simulink model "MIL4L3_SW6_V1_20220211"  (R2018b)
settings: Solver=FixedStepAuto  StartTime=0.0  StopTime=inf  FixedStep=0.001  RelTol=1e-3
PreLoadFcn:
  | A0_MILtest;
undefined symbols (not defined in the file or in its folder): Clb_ICADirect_LaneDisp_StateFive, Clb_ICADirect_LaneDisp_StateFour, Clb_ICADirect_LaneDisp_StateOne, Clb_ICADirect_LaneDisp_StateThree, Clb_ICADirect_LaneDisp_StateTwo, Clb_ICADirect_LaneDisp_StateZero, Clb_ICADirect_LaneDispSW, Clb_ICADirect_TrnLghtsCom_Switch, Clb_ICADirect_TrnLghtsCom_Value, Clb_ICADirect_TrnLghtsCrtl_Inhb, IMAP_Clb_ACU_Driver_Belt, IMAP_Clb_ACU_Driver_Belt_Over, IMAP_Clb_ACU_Passenger_Belt, IMAP_Clb_ACU_Passenger_Belt_Over, IMAP_Clb_ACU_RearLeft_Belt, IMAP_Clb_ACU_RearLeft_Belt_Over, IMAP_Clb_ACU_RearMiddle_Belt, IMAP_Clb_ACU_RearMiddle_Belt_Over, IMAP_Clb_ACU_RearRight_Belt, IMAP_Clb_ACU_RearRight_Belt_Over, IMAP_Clb_AEB_Switch, IMAP_Clb_AEB_Switch_Over, IMAP_Clb_ALC_TLC_Mode, IMAP_Clb_ALC_TLC_Mode_Over, IMAP_Clb_BCM_Battery_Voltage, IMAP_Clb_BCM_Battery_Voltage_Over, IMAP_Clb_BCM_BrakeLamp_State, IMAP_Clb_BCM_BrakeLamp_State_Over, IMAP_Clb_BCM_CHMSL_Status, IMAP_Clb_BCM_CHMSL_Status_Over, IMAP_Clb_BCM_Door_Lock_State, IMAP_Clb_BCM_Door_Lock_State_Over, IMAP_Clb_BCM_FrontWiper_State, IMAP_Clb_BCM_FrontWiper_State_Over, IMAP_Clb_BCM_FrontWiper_Switch, IMAP_Clb_BCM_FrontWiper_Switch_Over, IMAP_Clb_BCM_HazardLamp, IMAP_Clb_BCM_HazardLamp_Over, IMAP_Clb_BCM_HazardLamp_Switch, IMAP_Clb_BCM_HazardLamp_Switch_Over, IMAP_Clb_BCM_HighBeam_State, IMAP_Clb_BCM_HighBeam_State_Over, IMAP_Clb_BCM_Ignition_State, IMAP_Clb_BCM_Ignition_State_Over, IMAP_Clb_BCM_IHBC_Enabled, IMAP_Clb_BCM_IHBC_Enabled_Over, IMAP_Clb_BCM_Left_Light, IMAP_Clb_BCM_Left_Light_Over, IMAP_Clb_BCM_LeftTurn_Switch, IMAP_Clb_BCM_LeftTurn_Switch_Over, IMAP_Clb_BCM_LF_Door_State, IMAP_Clb_BCM_LF_Door_State_Over, IMAP_Clb_BCM_LowBeam_State, IMAP_Clb_BCM_LowBeam_State_Over, IMAP_Clb_BCM_LR_Door_State, IMAP_Clb_BCM_LR_Door_State_Over, IMAP_Clb_BCM_RF_Door_State, IMAP_Clb_BCM_RF_Door_State_Over, IMAP_Clb_BCM_Right_Light, IMAP_Clb_BCM_Right_Light_Over ... (+547)
libraries: CarMaker4SL x2153, simulink x292, dspstat3 x3, canmsglib x2, simulink_extras x1
(part 42 of 52)

== system MIL4L3_SW6_V1_20220211/CarMaker/VehicleControl/OMAP/OMAP1/Runnable_OMAP_10ms_sys/OMAP_Module/ACCS_Direct/ACCS_Define/ACC_State_Synthesis(ACC_SS)/If Action Subsystem3 ==
  ACT_Control_Signal : Inport
  Action Port : ActionPort  InitializeStates=reset  ActionType=else
  Bus Creator : BusCreator  Inputs=15
  Bus Selector1 : BusSelector  OutputSignals=ACCSve_g_ACC_TqReq_convert,ACCSve_d_ACC_TqFlag_convert,ACCSve_g_ACC_DecReq_convert,ACCSve_d_ACC_DecFlag_convert,ACCSve_d_ACC_State_convert,ACCSve_d_ACC_ESCDriveOff_convert,ACCSve_d_ACC_ESCHoldReq_convert,ACCSve_d_ACC_EPBReq_convert
  Constant5 : Constant  Value=0  OutDataTypeStr=uint8
  Data Type Conversion{,1..6} (7 alike) : DataTypeConversion  OutDataTypeStr=uint8
  Gain : Gain  OutDataTypeStr=single
  Signal Conversion : SignalConversion  OverrideOpt=off
  Subsystem : Subsystem
  Subsystem1 : Subsystem
  Subsystem2 : Subsystem
  Subsystem3 : Subsystem
  Subsystem5 : Subsystem
  Subsystem6 : Subsystem
  Control_Ouput : Outport
  wires:
  Bus Selector1/4 -> [ESC_Enable]  "<ACCSve_d_ACC_DecFlag_convert>"
  Bus Selector1/3 -> [ESC_DecTar]  "<ACCSve_g_ACC_DecReq_convert>"
  Bus Selector1/2 -> [EMS_Enable]  "<ACCSve_d_ACC_TqFlag_convert>"
  Bus Selector1/1 -> [EMS_DecTar]  "<ACCSve_g_ACC_TqReq_convert>"
  Data Type Conversion2/1 -> Bus Creator/11  "MDD_deceleration_type"
  Data Type Conversion1/1 -> Bus Creator/10  "MDD_Decelerationcontrol_request"
  Data Type Conversion/1 -> Bus Creator/8  "Powertrain_torquewheel_request"
  Subsystem6/1(TYPE_RAPPORT) -> Bus Creator/9  "TYPE_RAPPORT"
  [EMS_Enable] -> Data Type Conversion/1
  Signal Conversion/1 -> Control_Ouput/1
  Constant5/1 -> Bus Creator/12  "Power_steering_power_cut3F2"
  Gain/1 -> Bus Creator/5  "PotACCTqReq"
  [EMS_Enable] -> Subsystem5/2(In2)
  [EMS_DecTar] -> Subsystem5/1(In1)
  Subsystem3/1(Function_Acc_status) -> Bus Creator/6  "Function_Acc_status"
  Bus Selector1/5 -> Data Type Conversion3/1  "<ACCSve_d_ACC_State_convert>"
  Subsystem2/1(StAcvTqWhlPTPotReq) -> Bus Creator/4  "StAcvTqWhlPTPotReq"
  [ESC_Enable] -> Subsystem2/2(In2)
  Subsystem1/1(TminUpGear) -> Bus Creator/3  "TminUpGear"
  Subsystem/1(TminDownGear) -> Bus Creator/2  "TminDownGear"
  [EMS_Enable] -> Subsystem1/1(In1), Subsystem/1(In1), Subsystem2/1(In1)
  ACT_Control_Signal/1 -> Bus Selector1/1
  Bus Creator/1 -> Signal Conversion/1
  [ESC_DecTar] -> Bus Creator/1  "Deceleration_setpoint_device"
  [EMS_DecTar] -> Gain/1, Bus Creator/7  "ACCTqReq"
  [ESC_Enable] -> Data Type Conversion1/1
  [ESC_Enable] -> Data Type Conversion2/1
  Data Type Conversion3/1 -> Subsystem3/1(In1)
  [ESC_Hold] -> Data Type Conversion5/1
  [ESC_EPB] -> Data Type Conversion6/1
  [ESC_DriveOff] -> Data Type Conversion4/1
  Bus Selector1/6 -> [ESC_DriveOff]  "<ACCSve_d_ACC_ESCDriveOff_convert>"
  Bus Selector1/7 -> [ESC_Hold]  "<ACCSve_d_ACC_ESCHoldReq_convert>"
  Bus Selector1/8 -> [ESC_EPB]  "<ACCSve_d_ACC_EPBReq_convert>"
  Data Type Conversion4/1 -> Bus Creator/13  "OMAPve_y_ADAS_ESCDriveOff"
  Data Type Conversion5/1 -> Bus Creator/14  "OMAPve_y_ADAS_ESCHoldReq"
  Data Type Conversion6/1 -> Bus Creator/15  "OMAPve_y_ADAS_ACCRequestEPB"

== system MIL4L3_SW6_V1_20220211/CarMaker/VehicleControl/OMAP/OMAP1/Runnable_OMAP_10ms_sys/OMAP_Module/ACCS_Direct/ACCS_Define/Human_Machine_Interface(ACC_HMI)/Subsystem ==
  Distance : Inport
  CIPV_ID : Inport  Port=2
  ACC_State : Inport  Port=3
  Chart : Stateflow chart  TreatAsAtomicUnit=on
  Compare To Constant13 : simulink/Logic and Bit Operations/Compare To Constant  relop=>  const=0  OutDataTypeStr=boolean
  Compare To Constant14 : simulink/Logic and Bit Operations/Compare To Constant  relop===  const=4  OutDataTypeStr=boolean
  Compare To Constant16 : simulink/Logic and Bit Operations/Compare To Constant  relop===  const=7  OutDataTypeStr=boolean
  Compare To Constant17 : simulink/Logic and Bit Operations/Compare To Constant  relop===  const=8  OutDataTypeStr=boolean
  Compare To Constant18 : simulink/Logic and Bit Operations/Compare To Constant  relop===  const=5  OutDataTypeStr=boolean
  Constant : Constant  Value=5  OutDataTypeStr=uint8
  Constant1 : Constant  Value=0  OutDataTypeStr=uint8
  Logical Operator5 : Logic  Operator=OR  Inputs=4  AllPortsSameDT=off  OutDataTypeStr=boolean
  Switch : Switch  Criteria=u2 ~= 0
  Switch1 : Switch  Criteria=u2 ~= 0
  TARGET_POSITION : Outport
  TgDisp_Flag : Outport  Port=2
  wires:
  Distance/1 -> Chart/1(Distance)
  Chart/1(Value) -> Switch/1
  ACC_State/1 -> Compare To Constant16/1, Compare To Constant17/1, Compare To Constant14/1, Compare To Constant18/1
  Compare To Constant18/1 -> Logical Operator5/1
  Compare To Constant14/1 -> Logical Operator5/2
  Compare To Constant16/1 -> Logical Operator5/3
  Compare To Constant17/1 -> Logical Operator5/4
  Logical Operator5/1 -> Switch/2, Switch1/2
  Switch/1 -> TARGET_POSITION/1
  Constant/1 -> Switch/3
  Switch1/1 -> TgDisp_Flag/1
  CIPV_ID/1 -> Compare To Constant13/1
  Compare To Constant13/1 -> Switch1/1
  Constant1/1 -> Switch1/3

== system MIL4L3_SW6_V1_20220211/CarMaker/VehicleControl/OMAP/OMAP1/Runnable_OMAP_10ms_sys/OMAP_Module/ACCS_Direct/ACCS_Define/Human_Machine_Interface(ACC_HMI)/Subsystem9 ==
  ACC_State : Inport
  ACCICA_Flag : Inport  Port=2
  VelocitySet : Inport  Port=3
  Bus Creator : BusCreator  Inputs=4
  Bus Selector : BusSelector  OutputSignals=ACC_Vehicle_Icon_Display,ACC_Set_Speed_Display,ACC_DesiredHeadway_Icon_Basic,RVVACC_Vehiclespeed_request_type
  Constant : Constant  Value=0  OutDataTypeStr=uint16
  Multiport Switch : MultiPortSwitch  DataPortOrder=Specify indices  DataPortIndices={0,1,2,3,4,5,6,7,8,15}  DiagnosticForDefault=Warning
  Subsystem : Subsystem
  Subsystem1 : Subsystem
  Subsystem2 : Subsystem
  Subsystem3 : Subsystem
  Subsystem4 : Subsystem
  Subsystem5 : Subsystem
  Subsystem6 : Subsystem
  Subsystem7 : Subsystem
  Subsystem8 : Subsystem
  Switch : Switch  Criteria=u2 ~= 0
  Out1 : Outport
  wires:
  Subsystem/1(Out1) -> Multiport Switch/2, Multiport Switch/3
  Multiport Switch/1 -> Bus Selector/1
  ACC_State/1 -> Multiport Switch/1
  Subsystem2/1(Out1) -> Multiport Switch/5
  Subsystem1/1(Out1) -> Multiport Switch/4
  Subsystem3/1(Out1) -> Multiport Switch/6
  Subsystem4/1(Out1) -> Multiport Switch/7
  Subsystem5/1(Out1) -> Multiport Switch/8
  Subsystem6/1(Out1) -> Multiport Switch/9
  Subsystem7/1(Out1) -> Multiport Switch/10
  Subsystem8/1(Out1) -> Multiport Switch/11
  VelocitySet/1 -> Subsystem2/1(VelocitySet), Subsystem1/1(VelocitySet)
  ACCICA_Flag/1 -> Switch/2
  Constant/1 -> Switch/1
  Bus Creator/1 -> Out1/1
  Bus Selector/1 -> Switch/3  "<ACC_Vehicle_Icon_Display>"
  Bus Selector/2 -> Bus Creator/2  "<ACC_Set_Speed_Display>"
  Bus Selector/3 -> Bus Creator/3  "<ACC_DesiredHeadway_Icon_Basic>"
  Bus Selector/4 -> Bus Creator/4  "<RVVACC_Vehiclespeed_request_type>"
  Switch/1 -> Bus Creator/1  "ACC_Vehicle_Icon_Display"

== system MIL4L3_SW6_V1_20220211/CarMaker/VehicleControl/OMAP/OMAP1/Runnable_OMAP_10ms_sys/OMAP_Module/ACCS_Direct/ACCS_Define/Human_Machine_Interface(ACC_HMI)/Text_PopUp ==
  ACC_State : Inport
  ACCICA_Flag : Inport  Port=2
  ACCActive_Signal : Inport  Port=3
  go_request : Inport  Port=4
  ACC_DecReq : Inport  Port=5
  " Radar_Blocked" : Subsystem
  ACC_Activation_Unsatisfied : Subsystem
  ACC_Active : Subsystem
  ACC_Canceled : Subsystem
  ACC_Fault : Subsystem
  ACC_OFF : Subsystem
  ACC_ON : Subsystem
  ACC_go_request : Subsystem
  Cast : DataTypeConversion  OutDataTypeStr=uint8
  Constant : Constant  Value=0  OutDataTypeStr=uint16
  Constant1 : Constant  Value=0  OutDataTypeStr=uint16
  Gain : Gain
  Gain1 : Gain  Gain=10
  Gain2 : Gain  Gain=3
  Gain3 : Gain  Gain=8
  Gain4 : Gain  Gain=5
  Gain5 : Gain  Gain=2
  Gain6 : Gain  Gain=4
  Gain7 : Gain  Gain=7
  Gain9 : Gain  Gain=9
  Please_Take_Over_the_Car : Subsystem
  Please_Take_Over_the_Car_immediataly : Subsystem
  Radar_State : Constant  Value=2
  Switch{1..10} (10 alike) : Switch  Criteria=u2 > Threshold
  Switch11 : Switch  Criteria=u2 ~= 0
  Unit Delay1 : UnitDelay  SampleTime=-1
  gorequest : Gain  Gain=6
  For4F7 : Outport
  ForTJA : Outport  Port=2
  wires:
  ACC_ON/1(Out1) -> Gain/1
  Cast/1 -> " Radar_Blocked"/1(In1)
  " Radar_Blocked"/1(Out1) -> Gain5/1
  ACC_Fault/1(Out1) -> Gain2/1
  ACCActive_Signal/1 -> ACC_Activation_Unsatisfied/2(In2)
  ACC_Activation_Unsatisfied/1(Out1) -> Gain6/1
  ACC_Active/1(Out1) -> Gain4/1
  go_request/1 -> ACC_go_request/1(In1)
  ACC_go_request/1(<GoRequest>) -> gorequest/1
  Please_Take_Over_the_Car/1(Out1) -> Gain7/1
  ACC_State/1 -> ACC_OFF/1(In1), ACC_Canceled/1(In1), Please_Take_Over_the_Car/1(In1), ACC_Active/1(In1), ACC_Activation_Unsatisfied/1(In1), ACC_Fault/1(In1), ACC_ON/1(In1)
  Please_Take_Over_the_Car_immediataly/1(Out1) -> Gain3/1
  ACC_Canceled/1(Out1) -> Gain9/1
  ACC_OFF/1(Out1) -> Gain1/1
  Gain/1 -> Switch1/1, Switch1/2
  Gain5/1 -> Switch2/1, Switch2/2
  Gain2/1 -> Switch3/1, Switch3/2
  Gain6/1 -> Switch4/1, Switch4/2
  Gain4/1 -> Switch5/1, Switch5/2
  gorequest/1 -> Switch6/1, Switch6/2
  Gain7/1 -> Switch7/1, Switch7/2
  Gain3/1 -> Switch8/1, Switch8/2
  Gain9/1 -> Switch9/1, Switch9/2
  Constant/1 -> Switch1/3
  Switch1/1 -> Switch2/3
  Switch2/1 -> Switch3/3
  Switch3/1 -> Switch4/3
  Switch4/1 -> Switch5/3
  Switch5/1 -> Switch6/3
  Switch6/1 -> Switch7/3
  Switch7/1 -> Switch8/3
  Switch8/1 -> Switch9/3
  Gain1/1 -> Switch10/1, Switch10/2
  Switch9/1 -> Switch10/3
  Switch10/1 -> Unit Delay1/1, ForTJA/1, Switch11/3
  [ACCICA_Flag] -> Switch11/2
  Constant1/1 -> Switch11/1
  Switch11/1 -> For4F7/1
  [Text] -> ACC_ON/2(In2)
  Unit Delay1/1 -> [Text]
  [ACCICA_Flag] -> ACC_OFF/2(In2)
  ACCICA_Flag/1 -> [ACCICA_Flag]
  [ACCICA_Flag] -> ACC_ON/3(ACCICA_Flag)
  Radar_State/1 -> Cast/1
  ACC_DecReq/1 -> Please_Take_Over_the_Car_immediataly/1(ESC_DecTar)

== system MIL4L3_SW6_V1_20220211/CarMaker/VehicleControl/OMAP/OMAP1/Runnable_OMAP_10ms_sys/OMAP_Module/ICA_Direct_G59/ICA_Define/ICA_EPS/EPS_Ctr_Disable ==
  note: 默认值2
  stEPSCtlState : Inport
  Action Port : ActionPort  InitializeStates=reset  ActionType=else
  Constant : Constant  Value=0  OutDataTypeStr=single
  Constant1 : Constant  Value=0  OutDataTypeStr=uint16
  Constant2 : Constant  Value=OMAP_ICA_EPSCMDdisable  OutDataTypeStr=uint8
  Constant3 : Constant  Value=0  OutDataTypeStr=single
  Constant4 : Constant  Value=0  OutDataTypeStr=single
  MATLAB Function : MATLAB Function  TreatAsAtomicUnit=on
  stEPSCtlCMD : Outport
  LKA_TRQ_FACT_REQ : Outport  Port=2
  LKA_OR_LPA_REQ : Outport  Port=3
  angle1 : Outport  Port=4
  torque1 : Outport  Port=5
  wires:
  MATLAB Function/1(stEPSCtlCMD) -> stEPSCtlCMD/1
  stEPSCtlState/1 -> MATLAB Function/1(stEPSCtlState)
  Constant/1 -> LKA_TRQ_FACT_REQ/1  "LKA_TRQ_FACT_REQ"
  Constant1/1 -> LKA_OR_LPA_REQ/1  "LKA_OR_LPA_REQ"
  Constant3/1 -> angle1/1  "LKA_OR_LPA_REQ"
  Constant4/1 -> torque1/1  "LKA_OR_LPA_REQ"
  Constant2/1 -> MATLAB Function/2(ControlCMDdisable)

== system MIL4L3_SW6_V1_20220211/CarMaker/VehicleControl/OMAP/OMAP1/Runnable_OMAP_10ms_sys/OMAP_Module/ICA_Direct_G59/ICA_Define/ICA_EPS/EPS_Ctr_Enable ==
  note: 默认值2
  note: 默认值3
  note: 默认值4
  stEPSCtlState : Inport
  angle : Inport  Port=2
  torque : Inport  Port=3
  Action Port : ActionPort  InitializeStates=reset  ActionType=then
  Abs : Abs
  Constant : Constant  Value=OMAP_ICA_EPStrqfactor  OutDataTypeStr=single
  Constant1 : Constant  Value=0  OutDataTypeStr=uint16
  Constant2 : Constant  Value=OMAP_ICA_EPSCMDselect  OutDataTypeStr=uint8
  Constant3 : Constant  Value=OMAP_ICA_EPSCMDauthorized  OutDataTypeStr=uint8
  Constant4 : Constant  Value=OMAP_ICA_EPSCMDactive  OutDataTypeStr=uint8
  Constant5 : Constant  Value=OMAP_ICA_EPStrqfactorRate  OutDataTypeStr=single
  Gain : Gain  Gain=-1  OutDataTypeStr=single
  MATLAB Function : MATLAB Function  TreatAsAtomicUnit=on
  Rate Limiter Dynamic : simulink/Discontinuities/Rate Limiter Dynamic
      settings: SourceProductName=Simulink
  stEPSCtlCMD : Outport
  LKA_TRQ_FACT_REQ : Outport  Port=2
  LKA_OR_LPA_REQ : Outport  Port=3
  angle1 : Outport  Port=4
  torque1 : Outport  Port=5
  wires:
  stEPSCtlState/1 -> MATLAB Function/1(stEPSCtlState)
  MATLAB Function/1(stEPSCtlCMD) -> stEPSCtlCMD/1
  Rate Limiter Dynamic/1 -> LKA_TRQ_FACT_REQ/1  "LKA_TRQ_FACT_REQ"
  Constant1/1 -> LKA_OR_LPA_REQ/1  "LKA_OR_LPA_REQ"
  angle/1 -> angle1/1
  torque/1 -> torque1/1
  Constant2/1 -> MATLAB Function/2(EPSCMDselect)
  Constant3/1 -> MATLAB Function/3(EPSCMDauthorized)
  Constant4/1 -> MATLAB Function/4(EPSCMDactive)
  Constant/1 -> Rate Limiter Dynamic/2  "LKA_TRQ_FACT_REQ"
  Constant5/1 -> Abs/1  "LKA_TRQ_FACT_REQ"
  Abs/1 -> Gain/1, Rate Limiter Dynamic/1
  Gain/1 -> Rate Limiter Dynamic/3

== system MIL4L3_SW6_V1_20220211/CarMaker/VehicleControl/OMAP/OMAP1/Runnable_OMAP_10ms_sys/OMAP_Module/ICA_Direct_G59/ICA_Define/Subsystem1/Dspl ==
  note: 0是运动，1是静止
  note: 0 ：可以从降级回到正常，
      | 1 ：不可以从降级回到正常
  TxHndOff : Inport
  Dspl_stTkOvStChk : Inport  Port=2
  Dspl_facmL0Ql : Inport  Port=3
  Dspl_facmR0Ql : Inport  Port=4
  Dspl_stVehSty : Inport  Port=5
  Dspl_facmL0Type : Inport  Port=6
  Dspl_facmR0Type : Inport  Port=7
  Dspl_stTHState : Inport  Port=8
  Dspl_bsFromFMCMsg : Inport  Port=9
  Dspl_stTHFKeyState : Inport  Port=10
  DsplPrcs_CIb : Inport  Port=11
  Dspl_tfAddVocCmd : Inport  Port=12
  DsplPrcs_dDgrdIconWarnflag : Inport  Port=13
  DsplPrcs_stSWALimFlg : Inport  Port=14
  Dspl_stturn_lightState : Inport  Port=15
  Dspl_stTLC_ALCmodeSW : Inport  Port=16
  Dspl_stLC_SpdCndtFlg : Inport  Port=17
  Bus Selector5 : BusSelector  OutputSignals=TH_HMIClb_tiHndOffTxtWarnT_C,TH_HMIClb_tiDgrdVocWarnDurT_C,TH_HMIClb_tiHndOffVocWarnT_C,TH_HMIClb_tiTxtLimT_C,TH_HMIClb_tiDgrdIconWarnHiDurT_C,TH_HMIClb_tiDgrdIconWarnLoDurT_C,TH_HMIClb_tiSWALimFlgDetT_C,TH_HMIClb_tiCalcPer_C
  Data Type Conversion{,1..6} (7 alike) : DataTypeConversion  OutDataTypeStr=uint16
  DsplPrcs : Subsystem
  TimePrcs : Subsystem
  Dspl_stTxtDspl : Outport
  Dspl_stICAIcon : Outport  Port=2
  Dspl_stLaneDspl : Outport  Port=3
  Dspl_stL0DispType : Outport  Port=4
  Dspl_stR0DispType : Outport  Port=5
  Dspl_stVocDspl : Outport  Port=6
  Dspl_stHWAmode : Outport  Port=7
  Dspl_bsMon : Outport  Port=8
  wires:
  Dspl_stTHState/1 -> DsplPrcs/7(DsplPrcs_stTHState)
  Dspl_stTHFKeyState/1 -> DsplPrcs/9(DsplPrcs_stTHFKeyState)
  Dspl_bsFromFMCMsg/1 -> DsplPrcs/8(DsplPrcs_bsFromFMCMsg)
  Data Type Conversion/1 -> Dspl_stTxtDspl/1
  Data Type Conversion1/1 -> Dspl_stICAIcon/1
  Data Type Conversion2/1 -> Dspl_stLaneDspl/1
  DsplPrcs/6(DsplPrcs_stVocDspl) -> Data Type Conversion5/1
  DsplPrcs/1(DsplPrcs_stTxtDspl) -> Data Type Conversion/1
  DsplPrcs/2(DsplPrcs_stICAIcon) -> Data Type Conversion1/1
  Data Type Conversion5/1 -> Dspl_stVocDspl/1
  DsplPrcs/8(DsplPrcs_bsMon) -> Dspl_bsMon/1
  DsplPrcs_CIb/1 -> Bus Selector5/1
  TimePrcs/2(TimePrcs_dDgrdVocWarnDurnum) -> DsplPrcs/18(DsplPrcs_dDgrdVocWarnDurnum)
  TimePrcs/3(TimePrcs_dHndOffVocWarnnum) -> DsplPrcs/19(DsplPrcs_dHndOffVocWarnnum)
  TimePrcs/1(TimePrcs_dHndOffTxtWarnnum) -> DsplPrcs/17(DsplPrcs_dHndOffTxtWarnnum)
  TimePrcs/4(TimePrcs_dTxtLimnum) -> DsplPrcs/20(DsplPrcs_dTxtLimnum)
  Bus Selector5/3 -> TimePrcs/3(TimePrcs_tiHndOffVocWarnT_C)  "<TH_HMIClb_tiHndOffVocWarnT_C>"
  Bus Selector5/8 -> TimePrcs/8(TimePrcs_tiCalcPer_C)  "<TH_HMIClb_tiCalcPer_C>"
  Bus Selector5/4 -> TimePrcs/4(TimePrcs_tiTxtLimT_C)  "<TH_HMIClb_tiTxtLimT_C>"
  Bus Selector5/1 -> TimePrcs/1(TimePrcs_tiHndOffTxtWarnT_C)  "<TH_HMIClb_tiHndOffTxtWarnT_C>"
  Bus Selector5/2 -> TimePrcs/2(TimePrcs_tiDgrdVocWarnDurT_C)  "<TH_HMIClb_tiDgrdVocWarnDurT_C>"
  TxHndOff/1 -> DsplPrcs/1(DsplPrcs_stStWhlHld)
  Dspl_facmL0Ql/1 -> DsplPrcs/3(DsplPrcs_facmL0Ql)
  Dspl_facmR0Ql/1 -> DsplPrcs/4(DsplPrcs_facmR0Ql)
  Dspl_stVehSty/1 -> DsplPrcs/10(DsplPrcs_stVehSty)
  Dspl_tfAddVocCmd/1 -> DsplPrcs/11(DsplPrcs_tfAddVocCmd)
  TimePrcs/5(TimePrcs_dDgrdIconWarnHiDurnum) -> DsplPrcs/21(DsplPrcs_dDgrdIconWarnHiDurnum)
  TimePrcs/6(TimePrcs_dDgrdIconWarnLoDurnum) -> DsplPrcs/22(DsplPrcs_dDgrdIconWarnLoDurnum)
  Bus Selector5/5 -> TimePrcs/5(TimePrcs_tiDgrdIconWarnHiDurT_C)  "<TH_HMIClb_tiDgrdIconWarnHiDurT_C>"
  Bus Selector5/6 -> TimePrcs/6(TimePrcs_tiDgrdIconWarnLoDurT_C)  "<TH_HMIClb_tiDgrdIconWarnLoDurT_C>"
  DsplPrcs_dDgrdIconWarnflag/1 -> DsplPrcs/13(DsplPrcs_dDgrdIconWarnflag)
  DsplPrcs_stSWALimFlg/1 -> DsplPrcs/12(DsplPrcs_stSWALimFlg)
  Bus Selector5/7 -> TimePrcs/7(TimePrcs_tiSWALimFlgDetT_C)  "<TH_HMIClb_tiSWALimFlgDetT_C>"
  TimePrcs/7(TimePrcs_tiSWALimFlgDetnum) -> DsplPrcs/23(DsplPrcs_tiSWALimFlgDetnum)
  Dspl_stTkOvStChk/1 -> DsplPrcs/2(DsplPrcs_stTkOvStChk)
  Dspl_facmL0Type/1 -> DsplPrcs/5(DsplPrcs_facmL0Type)
  Dspl_facmR0Type/1 -> DsplPrcs/6(DsplPrcs_facmR0Type)
  Data Type Conversion3/1 -> Dspl_stL0DispType/1
  Data Type Conversion4/1 -> Dspl_stR0DispType/1
  DsplPrcs/3(DsplPrcs_stLaneDspl) -> Data Type Conversion2/1
  DsplPrcs/4(DsplPrcs_stL0DispType) -> Data Type Conversion3/1
  DsplPrcs/5(DsplPrcs_stR0DispType) -> Data Type Conversion4/1
  Dspl_stturn_lightState/1 -> DsplPrcs/14(DsplPrcs_stturn_lightState)
  Dspl_stTLC_ALCmodeSW/1 -> DsplPrcs/15(DsplPrcs_stTLC_ALCmodeSW)
  Dspl_stLC_SpdCndtFlg/1 -> DsplPrcs/16(DsplPrcs_stLC_SpdCndtFlg)
  DsplPrcs/7(DsplPrcs_stHWAmode) -> Data Type Conversion6/1
  Data Type Conversion6/1 -> Dspl_stHWAmode/1

== system MIL4L3_SW6_V1_20220211/CarMaker/VehicleControl/OMAP/OMAP1/Runnable_OMAP_10ms_sys/OMAP_Module/ICA_Direct_G59/ICA_Define/Subsystem1/Subsystem ==
  Vehicle_Line_Display_Org : Inport
  LCRMode : Inport  Port=2
  High_Time : Inport  Port=3
  Low_Time : Inport  Port=4
  ISA_Value : Inport  Port=5
  ISA_Type : Inport  Port=6
  THMode : Inport  Port=7
  LC_Scene : Inport  Port=8
  Compare To Constant : simulink/Logic and Bit Operations/Compare To Constant  relop===  const=uint16(4)  OutDataTypeStr=boolean
  Compare To Constant1 : simulink/Logic and Bit Operations/Compare To Constant  relop===  const=uint16(2)  OutDataTypeStr=boolean
  Compare To Constant2 : simulink/Logic and Bit Operations/Compare To Constant  relop===  const=uint16(3)  OutDataTypeStr=boolean
  Constant4 : Constant  Value=0  OutDataTypeStr=uint16
  Constant5 : Constant  Value=0  OutDataTypeStr=uint16
  Constant6 : Constant  Value=0  OutDataTypeStr=uint16
  Data Type Conversion : DataTypeConversion  OutDataTypeStr=uint16
  Data Type Conversion1 : DataTypeConversion  OutDataTypeStr=uint16
  Gain : Gain  Gain=100
  Gain1 : Gain  Gain=100
  Logical Operator1 : Logic  Operator=OR  AllPortsSameDT=off  OutDataTypeStr=boolean
  MATLAB Function : MATLAB Function  TreatAsAtomicUnit=on
  Subsystem : Subsystem
  Switch{1..3,6} (4 alike) : Switch  Criteria=u2 > Threshold
  TSR_Version_Only_Sign_Type : Outport
  Vehicle_Line_Display : Outport  Port=2
  ISA Value : Outport  Port=3
  wires:
  Vehicle_Line_Display_Org/1 -> Vehicle_Line_Display/1
  Compare To Constant/1 -> Switch1/2
  MATLAB Function/1(TSR_Version_Only_Sign_Type) -> Switch2/1, Switch1/1
  Switch1/1 -> TSR_Version_Only_Sign_Type/1
  Subsystem/1(Signal) -> Switch2/2
  Constant5/1 -> Switch2/3
  Switch2/1 -> Switch3/1
  Constant6/1 -> Switch3/3
  Switch3/1 -> Switch1/3
  Logical Operator1/1 -> Switch3/2
  High_Time/1 -> Gain/1
  Low_Time/1 -> Gain1/1
  Gain/1 -> Data Type Conversion/1
  Gain1/1 -> Data Type Conversion1/1
  Data Type Conversion/1 -> Subsystem/1(HiDurnum)
  Data Type Conversion1/1 -> Subsystem/2(LoDurnum)
  THMode/1 -> [THMode], Compare To Constant/1
  ISA_Value/1 -> Switch6/1, Switch6/2
  Constant4/1 -> Switch6/3
  Switch6/1 -> ISA Value/1
  LC_Scene/1 -> MATLAB Function/2(LC_Scene)
  [THMode] -> MATLAB Function/1(TH_Mode)
  LCRMode/1 -> [stLCRMode], Compare To Constant1/1, Compare To Constant2/1
  Compare To Constant1/1 -> Logical Operator1/1
  Compare To Constant2/1 -> Logical Operator1/2
  [stLCRMode] -> MATLAB Function/3(stLCRMode)

== system MIL4L3_SW6_V1_20220211/CarMaker/VehicleControl/OMAP/OMAP1/Runnable_OMAP_10ms_sys/OMAP_Module/ICA_Direct_G59/ICA_Define/Subsystem1/Subsystem1 ==
  note: 标定开关Calib_ICADirect_TrnLghtsCom_Switch默认值为1，走ICA_Direct内部判断
      | 标定值为0时，通过标定值Calib_ICADirect_TrnLghtsCom_Value来自主选择输出的值
  LCRMode : Inport
  Constant : Constant  OutDataTypeStr=uint16
  Constant1 : Constant  Value=2  OutDataTypeStr=uint16
  Constant2 : Constant  Value=0  OutDataTypeStr=uint16
  Constant3 : Constant  Value=Clb_ICADirect_TrnLghtsCom_Switch  OutDataTypeStr=uint16
  Constant4 : Constant  Value=Clb_ICADirect_TrnLghtsCom_Value  OutDataTypeStr=uint16
  Index Vector : MultiPortSwitch  DataPortOrder=Specify indices  DataPortIndices={2,3,0}  OutDataTypeStr=uint16
  Switch : Switch  Criteria=u2 > Threshold  OutDataTypeStr=uint16
  TurnLightsCmd : Outport
  wires:
  LCRMode/1 -> Index Vector/1
  Index Vector/1 -> Switch/1
  Constant/1 -> Index Vector/2
  Constant1/1 -> Index Vector/3
  Constant2/1 -> Index Vector/4
  Constant3/1 -> Switch/2
  Constant4/1 -> Switch/3
  Switch/1 -> TurnLightsCmd/1

== system MIL4L3_SW6_V1_20220211/CarMaker/VehicleControl/OMAP/OMAP1/Runnable_OMAP_10ms_sys/OMAP_Module/ICA_Direct_G59/ICA_Define/TH_HMIClb/ISA_TYPE ==
  In2 : Inport
  Switch : Switch  Criteria=u2 ~= 0  OutDataTypeStr=uint16
  tmp : Constant  Value=0  OutDataTypeStr=uint16
  Out1 : Outport
  wires:
  In2/1 -> Switch/2, Switch/1
  Switch/1 -> Out1/1
  tmp/1 -> Switch/3

== system MIL4L3_SW6_V1_20220211/CarMaker/VehicleControl/OMAP/OMAP1/Runnable_OMAP_10ms_sys/OMAP_Module/ICA_Direct_G59/ICA_Define/TH_HMIClb/ISA_Value ==
  In2 : Inport
  Switch : Switch  Criteria=u2 ~= 0  OutDataTypeStr=uint16
  tmp : Constant  Value=0  OutDataTypeStr=uint16
  Out1 : Outport
  wires:
  tmp/1 -> Switch/3
  Switch/1 -> Out1/1
  In2/1 -> Switch/1, Switch/2

== system MIL4L3_SW6_V1_20220211/CarMaker/VehicleControl/OMAP/OMAP1/Runnable_OMAP_10ms_sys/OMAP_Module/ICA_Direct_G59/ICA_Define/TH_HMIClb/LCScene_tmp ==
  In2 : Inport
  Switch : Switch  Criteria=u2 ~= 0  OutDataTypeStr=uint16
  tmp : Constant  Value=0  OutDataTypeStr=uint16
  Out1 : Outport
  wires:
  In2/1 -> Switch/2, Switch/1
  Switch/1 -> Out1/1
  tmp/1 -> Switch/3

== system MIL4L3_SW6_V1_20220211/CarMaker/VehicleControl/OMAP/OMAP1/Runnable_OMAP_10ms_sys/OMAP_Module/ICA_Direct_G59/ICA_Define/TH_HMIClb/Mode_tmp ==
  In2 : Inport
  Switch : Switch  Criteria=u2 ~= 0  OutDataTypeStr=uint16
  tmp : Constant  Value=0  OutDataTypeStr=uint16
  Out1 : Outport
  wires:
  tmp/1 -> Switch/3
  Switch/1 -> Out1/1
  In2/1 -> Switch/1, Switch/2

== system MIL4L3_SW6_V1_20220211/CarMaker/VehicleControl/OMAP/OMAP1/Runnable_OMAP_10ms_sys/OMAP_Module/ICA_Direct_G59/ICA_Define/TH_HMIClb/TH_HMIClb_tiDgrdIconWarnHiDurT_C ==
  In2 : Inport
  Constant : Constant  Value=TH_HMIClb_tiDgrdIconWarnHiDurT_C  OutDataTypeStr=single
  Switch : Switch  Criteria=u2 ~= 0  OutDataTypeStr=single
  Out1 : Outport
  wires:
  Constant/1 -> Switch/3
  Switch/1 -> Out1/1
  In2/1 -> Switch/1, Switch/2

== system MIL4L3_SW6_V1_20220211/CarMaker/VehicleControl/OMAP/OMAP1/Runnable_OMAP_10ms_sys/OMAP_Module/ICA_Direct_G59/ICA_Define/TH_HMIClb/TH_HMIClb_tiDgrdIconWarnLoDurT_C ==
  In2 : Inport
  Constant : Constant  Value=TH_HMIClb_tiDgrdIconWarnLoDurT_C  OutDataTypeStr=single
  Switch : Switch  Criteria=u2 ~= 0  OutDataTypeStr=single
  Out1 : Outport
  wires:
  In2/1 -> Switch/2, Switch/1
  Switch/1 -> Out1/1
  Constant/1 -> Switch/3

== system MIL4L3_SW6_V1_20220211/CarMaker/VehicleControl/OMAP/OMAP1/Runnable_OMAP_10ms_sys/OMAP_Module/ICA_Direct_G59/ICA_Define/TH_HMIClb/TH_HMIClb_tiDgrdVocWarnDurT_C ==
  In2 : Inport
  Switch : Switch  Criteria=u2 ~= 0  OutDataTypeStr=single
  TH_MIN_SPEED_UPPER 1 : Constant  Value=TH_HMIClb_tiDgrdVocWarnDurT_C  OutDataTypeStr=single
  Out1 : Outport
  wires:
  In2/1 -> Switch/2, Switch/1
  Switch/1 -> Out1/1
  TH_MIN_SPEED_UPPER 1/1 -> Switch/3

== system MIL4L3_SW6_V1_20220211/CarMaker/VehicleControl/OMAP/OMAP1/Runnable_OMAP_10ms_sys/OMAP_Module/ICA_Direct_G59/ICA_Define/TH_HMIClb/TH_HMIClb_tiHndOffTxtWarnT_C  ==
  In2 : Inport
  Switch : Switch  Criteria=u2 ~= 0  OutDataTypeStr=single
  TH_MIN_SPEED_UPPER 1 : Constant  Value=TH_HMIClb_tiHndOffTxtWarnT_C  OutDataTypeStr=single
  Out1 : Outport
  wires:
  In2/1 -> Switch/2, Switch/1
  Switch/1 -> Out1/1
  TH_MIN_SPEED_UPPER 1/1 -> Switch/3

== system MIL4L3_SW6_V1_20220211/CarMaker/VehicleControl/OMAP/OMAP1/Runnable_OMAP_10ms_sys/OMAP_Module/ICA_Direct_G59/ICA_Define/TH_HMIClb/TH_HMIClb_tiHndOffVocWarnT_C ==
  In2 : Inport
  Switch : Switch  Criteria=u2 ~= 0  OutDataTypeStr=single
  TH_MIN_SPEED_UPPER 1 : Constant  Value=TH_HMIClb_tiHndOffVocWarnT_C  OutDataTypeStr=single
  Out1 : Outport
  wires:
  TH_MIN_SPEED_UPPER 1/1 -> Switch/3
  Switch/1 -> Out1/1
  In2/1 -> Switch/1, Switch/2

== system MIL4L3_SW6_V1_20220211/CarMaker/VehicleControl/OMAP/OMAP1/Runnable_OMAP_10ms_sys/OMAP_Module/ICA_Direct_G59/ICA_Define/TH_HMIClb/TH_HMIClb_tiSWALimFlgDetT_C ==
  In2 : Inport
  Switch : Switch  Criteria=u2 ~= 0  OutDataTypeStr=single
  TH_HMIClb_tiSWALimFlgDetT_C : Constant  Value=TH_HMIClb_tiSWALimFlgDetT_C  OutDataTypeStr=single
  Out1 : Outport
  wires:
  TH_HMIClb_tiSWALimFlgDetT_C/1 -> Switch/3
  Switch/1 -> Out1/1
  In2/1 -> Switch/1, Switch/2

== system MIL4L3_SW6_V1_20220211/CarMaker/VehicleControl/OMAP/OMAP1/Runnable_OMAP_10ms_sys/OMAP_Module/ICA_Direct_G59/ICA_Define/TH_HMIClb/TH_HMIClb_tiTxtLimT_C ==
  In2 : Inport
  Constant : Constant  Value=TH_HMIClb_tiTxtLimT_C  OutDataTypeStr=single
  Switch : Switch  Criteria=u2 ~= 0  OutDataTypeStr=single
  Out1 : Outport
  wires:
  In2/1 -> Switch/2, Switch/1
  Switch/1 -> Out1/1
  Constant/1 -> Switch/3

== system MIL4L3_SW6_V1_20220211/CarMaker/VehicleControl/Function/LKA/LKAS1/LL/LL Inputs Mapping/bsLaneInfo/LanesReconstruct /RoadSide Offset/CrvDvtR0C0 ==
  offset : Inport
  <R0_C0> : Inport  Port=2
  <R0_Type> : Inport  Port=3
  Add1 : Sum  Inputs=+-  OutDataTypeStr=single
  Average Filter (AvrgFlt)1 : Subsystem
      mask Display:
      | port_label('input', 1, 'In');
      | port_label('input', 2, 'PtsNum');
      | port_label('output', 1, 'Out');
      | color('blue');
      | text(0.98,0.9,'VCDC Block','horizontalAlignment','right');
      | color('black');
      | text(0.5,0.55,'Average Filter','horizontalAlignment','center');
      | text(0.5,0.4,'(AvrgFlt)','horizontalAlignment','center');
  Compare To Constant1 : simulink/Logic and Bit Operations/Compare To Constant  relop===  const=10  OutDataTypeStr=boolean
  PtsNum1 : Constant  Value=10  OutDataTypeStr=single
  Switch1 : Switch  Criteria=u2 > Threshold
  R0_C0 : Outport
  wires:
  Average Filter (AvrgFlt)1/1(Out) -> R0_C0/1  "R0_C0"
  <R0_Type>/1 -> Compare To Constant1/1
  Compare To Constant1/1 -> Switch1/2
  offset/1 -> Add1/2
  Add1/1 -> Switch1/1
  <R0_C0>/1 -> Switch1/3, Add1/1
  Switch1/1 -> Average Filter (AvrgFlt)1/1(In)
  PtsNum1/1 -> Average Filter (AvrgFlt)1/2(PtsNum)

== system MIL4L3_SW6_V1_20220211/CarMaker/VehicleControl/Function/LKA/LKAS1/LL/LL Inputs Mapping/bsLaneInfo/LanesReconstruct /RoadSide Offset/HdAgCompL0C1 ==
  LL_CompHdAg_C : Inport
  L0_Q : Inport  Port=2
  L0_C1 : Inport  Port=3
  Add : Sum
  Compare To Constant1 : simulink/Logic and Bit Operations/Compare To Constant  relop===  const=3  OutDataTypeStr=boolean
  Switch1 : Switch  Criteria=u2 > Threshold
  Out1 : Outport
  wires:
  Add/1 -> Switch1/1
  L0_C1/1 -> Add/2, Switch1/3
  LL_CompHdAg_C/1 -> Add/1
  Switch1/1 -> Out1/1  "L0_C1"
  L0_Q/1 -> Compare To Constant1/1
  Compare To Constant1/1 -> Switch1/2

== system MIL4L3_SW6_V1_20220211/CarMaker/VehicleControl/Function/LKA/LKAS1/LL/LL Inputs Mapping/bsLaneInfo/LanesReconstruct /RoadSide Offset/HdAgCompR0C1 ==
  LL_CompHdAg_C : Inport
  R0_Q : Inport  Port=2
  R0_C1 : Inport  Port=3
  Add : Sum
  Compare To Constant1 : simulink/Logic and Bit Operations/Compare To Constant  relop===  const=3  OutDataTypeStr=boolean
  Switch1 : Switch  Criteria=u2 > Threshold
  Out1 : Outport
  wires:
  Compare To Constant1/1 -> Switch1/2
  R0_Q/1 -> Compare To Constant1/1
  Switch1/1 -> Out1/1  "R0_C1"
  LL_CompHdAg_C/1 -> Add/1
  R0_C1/1 -> Switch1/3, Add/2
  Add/1 -> Switch1/1

== system MIL4L3_SW6_V1_20220211/CarMaker/VehicleControl/Function/LKA/LKAS1/LL/LL Inputs Mapping/bsLaneInfo/LanesReconstruct /RoadSide Offset/Road Width Calculation (RoadWCal) ==
  RoadWCal_L0Info : Inport
  RoadWCal_R0Info : Inport  Port=2
  Add : Sum
  Average Filter (AvrgFlt)1 : Subsystem
      mask Display:
      | port_label('input', 1, 'In');
      | port_label('input', 2, 'PtsNum');
      | port_label('output', 1, 'Out');
      | color('blue');
      | text(0.98,0.9,'VCDC Block','horizontalAlignment','right');
      | color('black');
      | text(0.5,0.55,'Average Filter','horizontalAlignment','center');
      | text(0.5,0.4,'(AvrgFlt)','horizontalAlignment','center');
  Bus Selector1 : BusSelector  OutputSignals=R0_C0,R0_Q
  Bus Selector3 : BusSelector  OutputSignals=L0_C0,L0_Q
  Compare To Constant : simulink/Logic and Bit Operations/Compare To Constant  relop=>=  const=2  OutDataTypeStr=boolean
  Compare To Constant1 : simulink/Logic and Bit Operations/Compare To Constant  relop=>=  const=2  OutDataTypeStr=boolean
  Delay : Delay  DelayLength=1  InitialCondition=0
  Gain : Gain  Gain=-1
  Logical Operator : Logic  AllPortsSameDT=off  OutDataTypeStr=boolean
  PtsNum1 : Constant  Value=10  OutDataTypeStr=single
  Saturation1 : Saturate  UpperLimit=5.5  LowerLimit=2.5
      settings: AttributesFormatString="Min = %<LowerLimit>  Max = %<UpperLimit>"
  Switch : Switch  Criteria=u2 > Threshold
  RoadWCal_lRoadW : Outport
  wires:
  RoadWCal_L0Info/1 -> Bus Selector3/1
  RoadWCal_R0Info/1 -> Bus Selector1/1
  Bus Selector3/1 -> Gain/1  "<L0_C0>"
  Bus Selector1/1 -> Add/2  "<R0_C0>"
  Gain/1 -> Add/1
  Add/1 -> Switch/1
  Bus Selector3/2 -> Compare To Constant/1  "<L0_Q>"
  Bus Selector1/2 -> Compare To Constant1/1  "<R0_Q>"
  Compare To Constant/1 -> Logical Operator/1
  Compare To Constant1/1 -> Logical Operator/2
  Logical Operator/1 -> Switch/2
  Delay/1 -> Switch/3
  PtsNum1/1 -> Average Filter (AvrgFlt)1/2(PtsNum)
  Switch/1 -> Average Filter (AvrgFlt)1/1(In)
  Average Filter (AvrgFlt)1/1(Out) -> Saturation1/1
  Saturation1/1 -> Delay/1, RoadWCal_lRoadW/1

== system MIL4L3_SW6_V1_20220211/CarMaker/VehicleControl/Function/LKA/LKAS1/LL/LL Inputs Mapping/bsLaneInfo/LanesReconstruct /RoadSide Offset/Subsystem ==
  offset : Inport
  <L0_C0> : Inport  Port=2
  <L0_Type> : Inport  Port=3
  Add : Sum  OutDataTypeStr=single
  Average Filter (AvrgFlt) : Subsystem
      mask Display:
      | port_label('input', 1, 'In');
      | port_label('input', 2, 'PtsNum');
      | port_label('output', 1, 'Out');
      | color('blue');
      | text(0.98,0.9,'VCDC Block','horizontalAlignment','right');
      | color('black');
      | text(0.5,0.55,'Average Filter','horizontalAlignment','center');
      | text(0.5,0.4,'(AvrgFlt)','horizontalAlignment','center');
  Compare To Constant : simulink/Logic and Bit Operations/Compare To Constant  relop===  const=10  OutDataTypeStr=boolean
  PtsNum : Constant  Value=10  OutDataTypeStr=single
  Switch : Switch  Criteria=u2 > Threshold
  L0_C0 : Outport
  wires:
  Add/1 -> Switch/1
  PtsNum/1 -> Average Filter (AvrgFlt)/2(PtsNum)
  <L0_C0>/1 -> Switch/3, Add/1
  offset/1 -> Add/2
  Switch/1 -> Average Filter (AvrgFlt)/1(In)
  <L0_Type>/1 -> Compare To Constant/1
  Compare To Constant/1 -> Switch/2
  Average Filter (AvrgFlt)/1(Out) -> L0_C0/1  "L0_C0"

== system MIL4L3_SW6_V1_20220211/CarMaker/VehicleControl/Function/LKA/LKAS1/LL/LLOn/LKA/Driver Torque Addition (DTA)/Subsystem/LowPass ==
  T : Inport
  u : Inport  Port=2
  dT : Inport  Port=3
  Add : Sum  Inputs=+-
  Add1 : Sum
  Add2 : Sum  OutDataTypeStr=single
  Divide : Product  Inputs=*/
  Divide1 : Product  Inputs=**
  Memory3 : Memory  InheritSampleTime=on
  SWACmdSyn_tiSmplT_C4 : Constant  OutDataTypeStr=single
  Saturation : Saturate  UpperLimit=50  LowerLimit=0
      settings: AttributesFormatString="Min = %<LowerLimit>  Max = %<UpperLimit>"
  Switch : Switch  Criteria=u2 > Threshold  Threshold=1
  Unit Delay : UnitDelay  SampleTime=-1
  y : Outport
  wires:
  Switch/1 -> Unit Delay/1, y/1
  Memory3/1 -> Add2/2
  Saturation/1 -> Memory3/1, Switch/2
  Add2/1 -> Saturation/1
  SWACmdSyn_tiSmplT_C4/1 -> Add2/1
  Add1/1 -> Switch/1
  Unit Delay/1 -> Add1/2, Add/2
  Divide1/1 -> Add1/1
  Add/1 -> Divide1/2
  Divide/1 -> Divide1/1
  u/1 -> Add/1, Switch/3
  dT/1 -> Divide/1
  T/1 -> Divide/2

== system MIL4L3_SW6_V1_20220211/CarMaker/VehicleControl/Function/LKA/LKAS1/LL/LLOn/LKA/Driver Torque Addition (DTA)/Subsystem/LowPass1 ==
  T : Inport  OutDataTypeStr=single
  u : Inport  Port=2
  dT : Inport  Port=3  OutDataTypeStr=single
  Add : Sum  Inputs=+-
  Add1 : Sum
  Add2 : Sum  OutDataTypeStr=single
  Discrete Derivative : simulink/Discrete/Discrete Derivative  gainval=1.0  ICPrevScaledInput=0.0  OutMin=[]  OutMax=[]  OutDataTypeStr=single  OutputDataTypeScalingMode=single  OutDataType=fixdt(1, 16)  OutScaling=2^-10  DoSatur=off
  Divide : Product  Inputs=*/
  Divide1 : Product  Inputs=**
  Memory3 : Memory  InheritSampleTime=on
  SWACmdSyn_tiSmplT_C4 : Constant  OutDataTypeStr=single
  Saturation : Saturate  UpperLimit=50  LowerLimit=0
      settings: AttributesFormatString="Min = %<LowerLimit>  Max = %<UpperLimit>"
  Switch : Switch  Criteria=u2 > Threshold  Threshold=2
  Unit Delay : UnitDelay  SampleTime=-1
  y : Outport
  wires:
  T/1 -> Divide/2
  dT/1 -> Divide/1
  Discrete Derivative/1 -> Switch/3, Add/1
  Divide/1 -> Divide1/1
  Add/1 -> Divide1/2
  Divide1/1 -> Add1/1
  Unit Delay/1 -> Add/2, Add1/2
  Add1/1 -> Switch/1
  SWACmdSyn_tiSmplT_C4/1 -> Add2/1
  Add2/1 -> Saturation/1
  Saturation/1 -> Switch/2, Memory3/1
  Memory3/1 -> Add2/2
  Switch/1 -> y/1, Unit Delay/1
  u/1 -> Discrete Derivative/1

== system MIL4L3_SW6_V1_20220211/CarMaker/VehicleControl/Function/LKA/LKAS1/LL/LLOn/LKA/Driver Torque Addition (DTA)/Subsystem1/Moving Standard Deviation2 ==
  In1 : Inport
  Add2 : Sum  AccumDataTypeStr=uint8  OutDataTypeStr=single
  Constant : Constant  OutDataTypeStr=uint8
  Delay{,1..48} (49 alike) : Delay  DelayLength=1
  Divide : Product  Inputs=*/
  Memory3 : Memory  InheritSampleTime=on
  Mux : Mux  Inputs=50
  Saturation : Saturate  UpperLimit=50  LowerLimit=1
      settings: AttributesFormatString="Min = %<LowerLimit>  Max = %<UpperLimit>"
  Standard Deviation : dspstat3/Standard Deviation  run=off  directionMode=Entire input  dimension=2  reset_popup=None  roiEnable=off  roiType=Rectangles  roiPortion=Entire ROI  roiOutput=Individual statistics for each ROI  roiFlag=off
      settings: SourceProductName=DSP System Toolbox  SourceProductBaseCode=DS
  Sum of Elements : Sum  Inputs=+
  Out2 : Outport
  Out1 : Outport  Port=2
  wires:
  In1/1 -> Mux/1, Delay/1
  Delay2/1 -> Mux/4, Delay3/1
  Delay1/1 -> Mux/3, Delay2/1
  Mux/1 -> Standard Deviation/1, Sum of Elements/1
  Delay/1 -> Mux/2, Delay1/1
  Standard Deviation/1 -> Out1/1
  Delay3/1 -> Mux/5, Delay4/1
  Delay4/1 -> Mux/6, Delay5/1
  Delay7/1 -> Mux/9, Delay8/1
  Delay6/1 -> Mux/8, Delay7/1
  Delay5/1 -> Mux/7, Delay6/1
  Delay8/1 -> Delay9/1, Mux/10
  Delay18/1 -> Delay28/1, Mux/20
  Delay15/1 -> Mux/17, Delay16/1
  Delay16/1 -> Mux/18, Delay17/1
  Delay17/1 -> Mux/19, Delay18/1
  Delay14/1 -> Mux/16, Delay15/1
  Delay13/1 -> Mux/15, Delay14/1
  Delay10/1 -> Mux/12, Delay11/1
  Delay11/1 -> Mux/13, Delay12/1
  Delay12/1 -> Mux/14, Delay13/1
  Delay9/1 -> Mux/11, Delay10/1
  Delay28/1 -> Mux/21, Delay19/1
  Delay21/1 -> Mux/24, Delay22/1
  Delay20/1 -> Mux/23, Delay21/1
  Delay19/1 -> Mux/22, Delay20/1
  Delay22/1 -> Mux/25, Delay23/1
  Delay23/1 -> Mux/26, Delay24/1
  Delay26/1 -> Mux/29, Delay27/1
  Delay25/1 -> Mux/28, Delay26/1
  Delay24/1 -> Mux/27, Delay25/1
  Delay27/1 -> Delay38/1, Mux/30
  Delay37/1 -> Delay48/1, Mux/40
  Delay34/1 -> Mux/37, Delay35/1
  Delay35/1 -> Mux/38, Delay36/1
  Delay36/1 -> Mux/39, Delay37/1
  Delay33/1 -> Mux/36, Delay34/1
  Delay32/1 -> Mux/35, Delay33/1
  Delay29/1 -> Mux/32, Delay30/1
  Delay30/1 -> Mux/33, Delay31/1
  Delay31/1 -> Mux/34, Delay32/1
  Delay38/1 -> Mux/31, Delay29/1
  Delay48/1 -> Mux/41, Delay39/1
  Delay41/1 -> Mux/44, Delay42/1
  Delay40/1 -> Mux/43, Delay41/1
  Delay39/1 -> Mux/42, Delay40/1
  Delay42/1 -> Mux/45, Delay43/1
  Delay43/1 -> Mux/46, Delay44/1
  Delay46/1 -> Mux/49, Delay47/1
  Delay45/1 -> Mux/48, Delay46/1
  Delay44/1 -> Mux/47, Delay45/1
  Delay47/1 -> Mux/50
  Add2/1 -> Saturation/1
  Constant/1 -> Add2/1
  Memory3/1 -> Add2/2
  Sum of Elements/1 -> Divide/1
  Saturation/1 -> Divide/2, Memory3/1
  Divide/1 -> Out2/1

== system MIL4L3_SW6_V1_20220211/CarMaker/VehicleControl/Function/LKA/LKAS1/LL/LLOn/LKA/Driver Torque Addition (DTA)/Subsystem1/TickTime (TTime) ==
  Add2 : Sum  OutDataTypeStr=single
  Memory3 : Memory  InheritSampleTime=on
  Saturation : Saturate  UpperLimit=50  LowerLimit=0
      settings: AttributesFormatString="Min = %<LowerLimit>  Max = %<UpperLimit>"
  Out1 : Outport
  wires:
  Add2/1 -> Saturation/1
  Memory3/1 -> Add2/2
  Saturation/1 -> Out1/1, Memory3/1
  [LKA_SampleTime] -> Add2/1

== system MIL4L3_SW6_V1_20220211/CarMaker/VehicleControl/Function/LKA/LKAS1/LL/LLOn/LKA/LKA Exit Processing (LKAExPrcs)/Exit Time 2/Sum Condition1 ==
  Sample Time : Inport
  Time Exit 2 : Inport  Port=2
  Enable : EnablePort  StatesWhenEnabling=reset
      settings: AttributesFormatString=states = %<StatesWhenEnabling>
  Add1 : Sum  OutDataTypeStr=single
  Memory : Memory  InheritSampleTime=on
  Relational Operator : RelationalOperator  OutDataTypeStr=boolean  RndMeth=Nearest
  Saturation : Saturate  UpperLimit=10  LowerLimit=0
      settings: AttributesFormatString="Min = %<LowerLimit>  Max = %<UpperLimit>"
  Out : Outport  OutputWhenDisabled=reset  InitialOutput=0
      settings: AttributesFormatString=%<OutputWhenDisabled> = %<InitialOutput>
  wires:
  Saturation/1 -> Memory/1, Relational Operator/1
  Memory/1 -> Add1/2
  Add1/1 -> Saturation/1
  Sample Time/1 -> Add1/1
  Time Exit 2/1 -> Relational Operator/2
  Relational Operator/1 -> Out/1

== system MIL4L3_SW6_V1_20220211/CarMaker/VehicleControl/Function/LKA/LKAS1/LL/LLOn/LKA/LKA Exit Processing (LKAExPrcs)/Exit Time 3/Moving Standard Deviation1 ==
  In1 : Inport
  Delay{,1..48} (49 alike) : Delay  DelayLength=1
  Mux : Mux  Inputs=50
  Standard Deviation : dspstat3/Standard Deviation  run=off  directionMode=Entire input  dimension=2  reset_popup=None  roiEnable=off  roiType=Rectangles  roiPortion=Entire ROI  roiOutput=Individual statistics for each ROI  roiFlag=off
      settings: SourceProductName=DSP System Toolbox  SourceProductBaseCode=DS
  Out1 : Outport
  wires:
  Delay47/1 -> Mux/50
  Delay44/1 -> Delay45/1, Mux/47
  Delay45/1 -> Delay46/1, Mux/48
  Delay46/1 -> Delay47/1, Mux/49
  Delay43/1 -> Delay44/1, Mux/46
  Delay42/1 -> Delay43/1, Mux/45
  Delay39/1 -> Delay40/1, Mux/42
  Delay40/1 -> Delay41/1, Mux/43
  Delay41/1 -> Delay42/1, Mux/44
  Delay48/1 -> Delay39/1, Mux/41
  Delay38/1 -> Delay29/1, Mux/31
  Delay31/1 -> Delay32/1, Mux/34
  Delay30/1 -> Delay31/1, Mux/33
  Delay29/1 -> Delay30/1, Mux/32
  Delay32/1 -> Delay33/1, Mux/35
  Delay33/1 -> Delay34/1, Mux/36
  Delay36/1 -> Delay37/1, Mux/39
  Delay35/1 -> Delay36/1, Mux/38
  Delay34/1 -> Delay35/1, Mux/37
  Delay37/1 -> Mux/40, Delay48/1
  Delay27/1 -> Mux/30, Delay38/1
  Delay24/1 -> Delay25/1, Mux/27
  Delay25/1 -> Delay26/1, Mux/28
  Delay26/1 -> Delay27/1, Mux/29
  Delay23/1 -> Delay24/1, Mux/26
  Delay22/1 -> Delay23/1, Mux/25
  Delay19/1 -> Delay20/1, Mux/22
  Delay20/1 -> Delay21/1, Mux/23
  Delay21/1 -> Delay22/1, Mux/24
  Delay28/1 -> Delay19/1, Mux/21
  Delay9/1 -> Delay10/1, Mux/11
  Delay12/1 -> Delay13/1, Mux/14
  Delay11/1 -> Delay12/1, Mux/13
  Delay10/1 -> Delay11/1, Mux/12
  Delay13/1 -> Delay14/1, Mux/15
  Delay14/1 -> Delay15/1, Mux/16
  Delay17/1 -> Delay18/1, Mux/19
  Delay16/1 -> Delay17/1, Mux/18
  Delay15/1 -> Delay16/1, Mux/17
  Delay18/1 -> Mux/20, Delay28/1
  Delay8/1 -> Mux/10, Delay9/1
  Delay5/1 -> Delay6/1, Mux/7
  Delay6/1 -> Delay7/1, Mux/8
  Delay7/1 -> Delay8/1, Mux/9
  Delay4/1 -> Delay5/1, Mux/6
  Delay3/1 -> Delay4/1, Mux/5
  Standard Deviation/1 -> Out1/1
  Delay/1 -> Delay1/1, Mux/2
  Mux/1 -> Standard Deviation/1
  Delay1/1 -> Delay2/1, Mux/3
  Delay2/1 -> Delay3/1, Mux/4
  In1/1 -> Delay/1, Mux/1

== system MIL4L3_SW6_V1_20220211/CarMaker/VehicleControl/Function/LKA/LKAS1/LL/LLOn/LKA/LKA Exit Processing (LKAExPrcs)/Exit Time 3/Moving Standard Deviation2 ==
  In1 : Inport
  Delay{,1..48} (49 alike) : Delay  DelayLength=1
  Mux : Mux  Inputs=50
  Standard Deviation : dspstat3/Standard Deviation  run=off  directionMode=Entire input  dimension=2  reset_popup=None  roiEnable=off  roiType=Rectangles  roiPortion=Entire ROI  roiOutput=Individual statistics for each ROI  roiFlag=off
      settings: SourceProductName=DSP System Toolbox  SourceProductBaseCode=DS
  Out1 : Outport
  wires:
  In1/1 -> Mux/1, Delay/1
  Delay2/1 -> Mux/4, Delay3/1
  Delay1/1 -> Mux/3, Delay2/1
  Mux/1 -> Standard Deviation/1
  Delay/1 -> Mux/2, Delay1/1
  Standard Deviation/1 -> Out1/1
  Delay3/1 -> Mux/5, Delay4/1
  Delay4/1 -> Mux/6, Delay5/1
  Delay7/1 -> Mux/9, Delay8/1
  Delay6/1 -> Mux/8, Delay7/1
  Delay5/1 -> Mux/7, Delay6/1
  Delay8/1 -> Delay9/1, Mux/10
  Delay18/1 -> Delay28/1, Mux/20
  Delay15/1 -> Mux/17, Delay16/1
  Delay16/1 -> Mux/18, Delay17/1
  Delay17/1 -> Mux/19, Delay18/1
  Delay14/1 -> Mux/16, Delay15/1
  Delay13/1 -> Mux/15, Delay14/1
  Delay10/1 -> Mux/12, Delay11/1
  Delay11/1 -> Mux/13, Delay12/1
  Delay12/1 -> Mux/14, Delay13/1
  Delay9/1 -> Mux/11, Delay10/1
  Delay28/1 -> Mux/21, Delay19/1
  Delay21/1 -> Mux/24, Delay22/1
  Delay20/1 -> Mux/23, Delay21/1
  Delay19/1 -> Mux/22, Delay20/1
  Delay22/1 -> Mux/25, Delay23/1
  Delay23/1 -> Mux/26, Delay24/1
  Delay26/1 -> Mux/29, Delay27/1
  Delay25/1 -> Mux/28, Delay26/1
  Delay24/1 -> Mux/27, Delay25/1
  Delay27/1 -> Delay38/1, Mux/30
  Delay37/1 -> Delay48/1, Mux/40
  Delay34/1 -> Mux/37, Delay35/1
  Delay35/1 -> Mux/38, Delay36/1
  Delay36/1 -> Mux/39, Delay37/1
  Delay33/1 -> Mux/36, Delay34/1
  Delay32/1 -> Mux/35, Delay33/1
  Delay29/1 -> Mux/32, Delay30/1
  Delay30/1 -> Mux/33, Delay31/1
  Delay31/1 -> Mux/34, Delay32/1
  Delay38/1 -> Mux/31, Delay29/1
  Delay48/1 -> Mux/41, Delay39/1
  Delay41/1 -> Mux/44, Delay42/1
  Delay40/1 -> Mux/43, Delay41/1
  Delay39/1 -> Mux/42, Delay40/1
  Delay42/1 -> Mux/45, Delay43/1
  Delay43/1 -> Mux/46, Delay44/1
  Delay46/1 -> Mux/49, Delay47/1
  Delay45/1 -> Mux/48, Delay46/1
  Delay44/1 -> Mux/47, Delay45/1
  Delay47/1 -> Mux/50

== system MIL4L3_SW6_V1_20220211/CarMaker/VehicleControl/Function/LKA/LKAS1/LL/LLOn/LKA/LKA Exit Processing (LKAExPrcs)/Exit Time 3/Sum Condition ==
  In : Inport
  In1 : Inport  Port=2
  Enable : EnablePort  StatesWhenEnabling=reset
      settings: AttributesFormatString=states = %<StatesWhenEnabling>
  Add1 : Sum  OutDataTypeStr=single
  Memory : Memory  InheritSampleTime=on
  Relational Operator : RelationalOperator  OutDataTypeStr=boolean  RndMeth=Nearest
  Saturation : Saturate  UpperLimit=100  LowerLimit=0
      settings: AttributesFormatString="Min = %<LowerLimit>  Max = %<UpperLimit>"
  Out : Outport  OutputWhenDisabled=reset  InitialOutput=0
      settings: AttributesFormatString=%<OutputWhenDisabled> = %<InitialOutput>
  wires:
  Saturation/1 -> Memory/1, Relational Operator/1
  Memory/1 -> Add1/2
  Add1/1 -> Saturation/1
  In/1 -> Add1/1
  In1/1 -> Relational Operator/2
  Relational Operator/1 -> Out/1

== system MIL4L3_SW6_V1_20220211/CarMaker/VehicleControl/Function/LKA/LKAS1/LL/LLOn/LKA/LKA Exit Processing (LKAExPrcs)/Exit Time 3/Sum Condition1 ==
  In : Inport
  In1 : Inport  Port=2
  Enable : EnablePort  StatesWhenEnabling=reset
      settings: AttributesFormatString=states = %<StatesWhenEnabling>
  Add1 : Sum  OutDataTypeStr=single
  Memory : Memory  InheritSampleTime=on
  Relational Operator : RelationalOperator  OutDataTypeStr=boolean  RndMeth=Nearest
  Saturation : Saturate  UpperLimit=100  LowerLimit=0
      settings: AttributesFormatString="Min = %<LowerLimit>  Max = %<UpperLimit>"
  Out : Outport  OutputWhenDisabled=reset  InitialOutput=0
      settings: AttributesFormatString=%<OutputWhenDisabled> = %<InitialOutput>
  wires:
  Relational Operator/1 -> Out/1
  In1/1 -> Relational Operator/2
  In/1 -> Add1/1
  Add1/1 -> Saturation/1
  Memory/1 -> Add1/2
  Saturation/1 -> Relational Operator/1, Memory/1

== system MIL4L3_SW6_V1_20220211/CarMaker/VehicleControl/Function/LKA/LKAS1/LL/LLOn/LKA/LKA Motion Planning (LKAMP) /LKA Motion Planning Calculation (LKAMPCal)/Time Division (TDiv) ==
  TDiv_bsTDivInfoOut : Inport
  Add : Sum  OutDataTypeStr=uint16
  Constant : Constant  OutDataTypeStr=uint16  SampleTime=-1
  Constant19 : Constant  OutDataTypeStr=uint16  SampleTime=-1
  If : If  NumInputs=2  IfExpression=u1==u2
  Memory : Memory  InheritSampleTime=on
  Merge : Merge
  Saturation1 : Saturate  UpperLimit=100  LowerLimit=0  OutDataTypeStr=uint16
      settings: AttributesFormatString="Min = %<LowerLimit>  Max = %<UpperLimit>"
  if action 1 : Subsystem  TreatAsAtomicUnit=on
  if action 2 : Subsystem  TreatAsAtomicUnit=on
  Out1 : Outport
  wires:
  TDiv_bsTDivInfoOut/1 -> if action 1/1(In1)
  if action 1/1(Out1) -> Merge/2
  Merge/1 -> Out1/1
  if action 2/1(Out1) -> Merge/1
  If/1 -> if action 2/Action
  If/2 -> if action 1/Action
  Memory/1 -> Add/2
  Constant/1 -> Add/1
  Constant19/1 -> If/2
  Add/1 -> Memory/1, Saturation1/1
  Saturation1/1 -> If/1

== system MIL4L3_SW6_V1_20220211/CarMaker/VehicleControl/Function/LKA/LKAS1/LL/LLOn/LKA/LKA Motion Planning (LKAMP) /LKA Motion Planning Calculation (LKAMPCal)/Time Division (TDiv)1 ==
  TDiv_bsTDivInfoOut1 : Inport
  Add : Sum  OutDataTypeStr=uint16
  Constant : Constant  OutDataTypeStr=uint16  SampleTime=-1
  Constant19 : Constant  OutDataTypeStr=uint16  SampleTime=-1
  If : If  NumInputs=2  IfExpression=u1==u2
  Memory : Memory  InheritSampleTime=on
  Merge1 : Merge
  Saturation1 : Saturate  UpperLimit=100  LowerLimit=0  OutDataTypeStr=uint16
      settings: AttributesFormatString="Min = %<LowerLimit>  Max = %<UpperLimit>"
  if action 3 : Subsystem  TreatAsAtomicUnit=on
  if action 4 : Subsystem  TreatAsAtomicUnit=on
  Out2 : Outport
  wires:
  Merge1/1 -> Out2/1
  TDiv_bsTDivInfoOut1/1 -> if action 3/1(In1)
  if action 4/1(Out1) -> Merge1/1
  if action 3/1(Out1) -> Merge1/2
  If/2 -> if action 3/Action
  Saturation1/1 -> If/1
  Add/1 -> Saturation1/1, Memory/1
  Constant19/1 -> If/2
  Constant/1 -> Add/1
  Memory/1 -> Add/2
  If/1 -> if action 4/Action

== system MIL4L3_SW6_V1_20220211/CarMaker/VehicleControl/Function/LKA/LKAS1/LL/LLOn/LKA/LKA Motion Planning (LKAMP) /LKA Motion Planning Calculation (LKAMPCal)/Time Division (TDiv)2 ==
  TDiv_bsTDivInfoOut1 : Inport
  Add : Sum  OutDataTypeStr=uint16
  Constant : Constant  OutDataTypeStr=uint16  SampleTime=-1
  Constant19 : Constant  OutDataTypeStr=uint16  SampleTime=-1
  If : If  NumInputs=2  IfExpression=u1==u2
  Memory : Memory  InheritSampleTime=on
  Merge1 : Merge
  Saturation1 : Saturate  UpperLimit=100  LowerLimit=0  OutDataTypeStr=uint16
      settings: AttributesFormatString="Min = %<LowerLimit>  Max = %<UpperLimit>"
  if action 3 : Subsystem  TreatAsAtomicUnit=on
  if action 4 : Subsystem  TreatAsAtomicUnit=on
  Out2 : Outport
  wires:
  If/1 -> if action 4/Action
  Memory/1 -> Add/2
  Constant/1 -> Add/1
  Constant19/1 -> If/2
  Add/1 -> Memory/1, Saturation1/1
  Saturation1/1 -> If/1
  If/2 -> if action 3/Action
  if action 3/1(Out1) -> Merge1/2
  if action 4/1(Out1) -> Merge1/1
  TDiv_bsTDivInfoOut1/1 -> if action 3/1(In1)
  Merge1/1 -> Out2/1
